simulink model "ABS_CHO"  (R2023a)
settings: Solver=ode45  StartTime=0  StopTime=15  FixedStep=0.001  RelTol=1e-3  AbsTol=1e-6
libraries: simulink x19, dspsigops x7, Solver_SF x1
(part 1 of 2)
settings Model: ExtModeTrigMode=oneshot  Creator=jhu  LastModifiedBy=USER
settings SolverCC: AutoScaleAbsTol=off  AlgebraicLoopSolver=TrustRegion
settings DataIOCC: SaveFormat=Array  SignalLoggingSaveFormat=ModelDataLogs  ReturnWorkspaceOutputs=off  SignalLoggingName=sigsOut
settings OptimizationCC: BlockReduction=off  BooleanDataType=off  ExpressionDepthLimit=2147483647  LifeSpan=inf
settings DebuggingCC: SaveWithParameterizedLinksMsg=none  UnderspecifiedInitializationDetection=Classic  MergeDetectMultiDrivingBlocksExec=none  SignalResolutionControl=TryResolveAllWithWarning  MultiTaskDSMMsg=warning  MultiTaskCondExecSysMsg=none  FcnCallInpInsideContextMsg=warning  UnconnectedInputMsg=warning  UnconnectedOutputMsg=warning  UnconnectedLineMsg=warning  StateNameClashWarn=warning  SFUnexpectedBacktrackingDiag=warning  SFNoUnconditionalDefaultTransitionDiag=warning  SFExecutionAtInitializationDiag=none  ArithmeticOperatorsInVariantConditions=warning
settings HardwareCC: ProdBitPerPointer=32  ProdBitPerSizeT=32  ProdBitPerPtrDiffT=32  ProdLargestAtomicFloat=None  ProdIntDivRoundTo=Undefined  ProdEndianess=Unspecified  ProdWordSize=32  ProdHWDeviceType=32-bit Generic  TargetUnknown=on
settings ModelReferenceCC: PropagateSignalLabelsOutOfModel=off
settings SFSimCC: SimUseLocalCustomCode=off  CustomCodeUndefinedFunction=UseInterfaceOnly
settings RTWCC: TemplateMakefile=grt_vc.tmf  RTWUseLocalCustomCode=off
settings CodeAppCC: StateflowObjectComments=on
settings GRTTargetCC: TargetFcnLib=ansi_tfl_tmw.mat  TargetLangStandard=C89/C90 (ANSI)  CombineOutputUpdateFcns=off  GRTInterface=on
settings ConfigComp: CovMetricSettings=dw  CovSaveCumulativeToWorkspaceVar=on  CovSaveSingleToWorkspaceVar=on  CovExternalEMLEnable=off

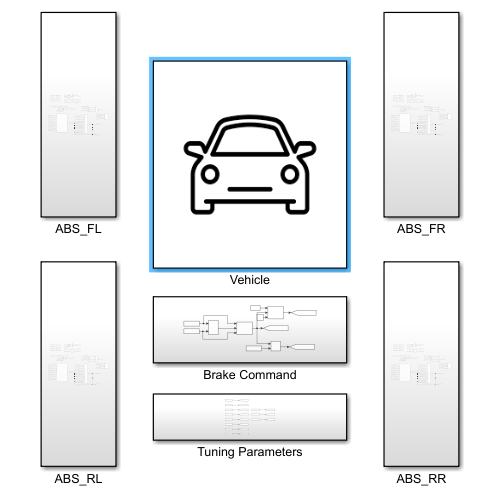
[thumbnail: Simulink's stored preview of the top-level diagram]
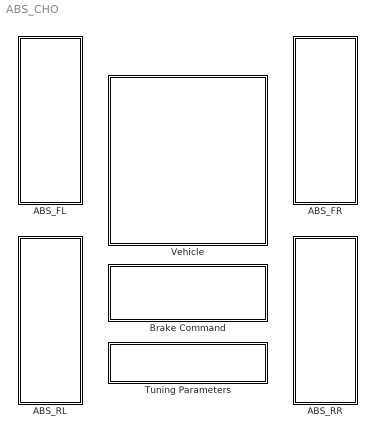
== system ABS_CHO ==
  ABS_FL : Subsystem
  ABS_FR : Subsystem
  ABS_RL : Subsystem
  ABS_RR : Subsystem
  Brake Command : Subsystem
  Tuning Parameters : Subsystem
  Vehicle : Subsystem
      mask Display: image('C:\Users\USER\Downloads\vehicle_icon.png'); % Use "Edit Image" on toolstrip to change.

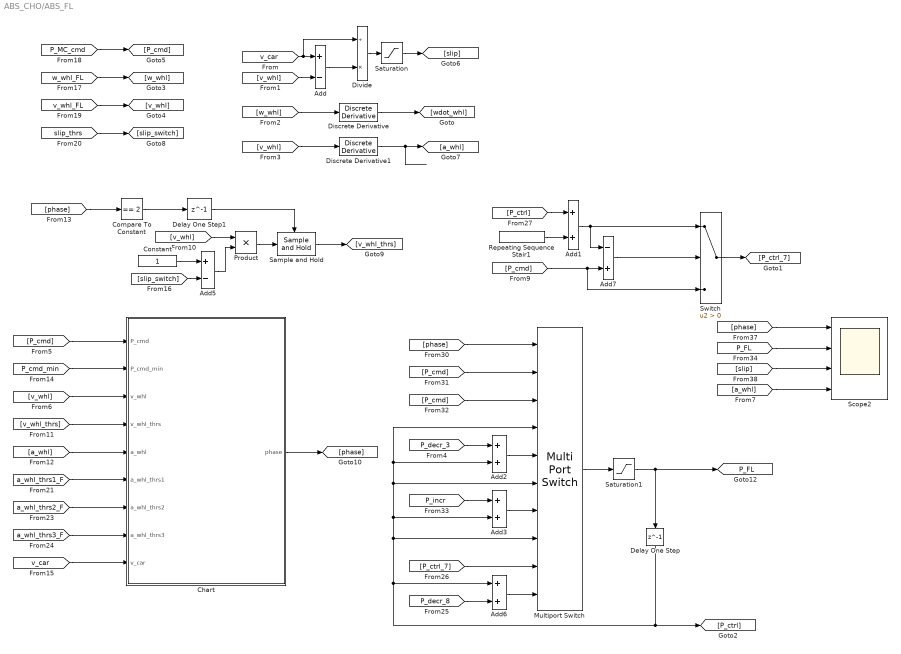
== system ABS_CHO/ABS_FL ==
  Add : Sum  Inputs=+-
  Add{1..3,6} (4 alike) : Sum
  Add5 : Sum  Inputs=+-
  Add7 : Sum  Inputs=-+
  Chart : Stateflow chart  TreatAsAtomicUnit=on
      settings: PortSchema="{\"entries\":[{\"content\":{\"sides\":[{\"content\":{\"connectorIds\":[\"In4\",\"In5\",\"In2\",\"In9\",\"In1\",\"In6\",\"In7\",\"In8\",\"In3\"]},\"type\":\"ConnectorPlacement.EquallySpacedRectSide\",\"uuid\":\"d1b40d47-5080-4bdb-9b64-2db0b8a6d570\"},{\"content\":{\"connectorIds\":[\"Out1\"],\"side\":\"RIGHT\"},\"type\":\"ConnectorPlacement.EquallySpacedRectSide\",\"uuid\":\"3562d231-244b-4945-a90c-51a654d62f0f\"},{\"content\":{\"side\":\"TOP\"},\"type\":\"ConnectorPlacement.EquallySpacedRectSide\",\"uuid\":\"6c914ffe-04dc-4ab2-bade-76d69248353c\"}]},\"type\":\"ConnectorPlacement.EquallySpacedConnector\",\"uuid\":\"36a59ec9-6bc3-461d-a020-c1da85e3b47f\"}],\"packageUris\":[\"http://schema.mathworks.com/mf0/Connector/R2020b\"],\"version\":\"1.0\"}"
  Compare To Constant : simulink/Logic and Bit Operations/Compare To Constant  relop===  const=2  OutDataTypeStr=boolean
  Constant : Constant
  Delay One Step : Delay  DelayLength=1  SampleTime=0.01
  Delay One Step1 : Delay  DelayLength=1  SampleTime=0.01
  Discrete Derivative : simulink/Discrete/Discrete Derivative  gainval=1.0  ICPrevScaledInput=0.0  OutMin=[]  OutMax=[]  OutDataType=fixdt(1, 16)  OutScaling=2^-10  DoSatur=off
  Discrete Derivative1 : simulink/Discrete/Discrete Derivative  gainval=1.0  ICPrevScaledInput=0.0  OutMin=[]  OutMax=[]  OutDataType=fixdt(1, 16)  OutScaling=2^-10  DoSatur=off
  Divide : Product  Inputs=/*
  Multiport Switch : MultiPortSwitch  DataPortOrder=Zero-based contiguous  Inputs=9  zeroidx=on  SaturateOnIntegerOverflow=off  InputSameDT=off
  Product : Product
  Repeating Sequence Stair1 : simulink/Sources/Repeating Sequence Stair  OutValues=[0.2 0].'  tsamp=0.01  OutMin=[]  OutMax=[]  OutDataTypeStr=double  OutputDataTypeScalingMode=double  OutDataType=fixdt(0,8)  ConRadixGroup=Best Precision: Vector-wise  OutScaling=2^-12
  Sample and Hold : dspsigops/Sample and Hold  trig=Rising edge  initCond=0  latchinput=off
  Saturation : Saturate  UpperLimit=1  LowerLimit=-1
  Saturation1 : Saturate  UpperLimit=30  LowerLimit=0
  Scope2 : Scope  NumInputPorts=4
  Switch : Switch  Criteria=u2 > Threshold  SaturateOnIntegerOverflow=off  InputSameDT=off
  tag scope: P_FL=global
  wires:
  Delay One Step/1 -> [P_ctrl], Add6/1, Multiport Switch/6, Add2/2, Multiport Switch/4, Add3/2, Multiport Switch/8
  Switch/1 -> [P_ctrl_7]
  Add7/1 -> Switch/2
  [P_cmd] -> Add7/2, Switch/3
  Add1/1 -> Add7/1, Switch/1
  Repeating Sequence Stair1/1 -> Add1/2
  [P_ctrl] -> Add1/1
  [v_car] -> Divide/1, Add/1
  [v_whl] -> Add/2
  Add/1 -> Divide/2
  Divide/1 -> Saturation/1
  Saturation/1 -> [slip]
  [w_whl] -> Discrete Derivative/1
  Discrete Derivative/1 -> [wdot_whl]
  [v_whl] -> Discrete Derivative1/1
  Discrete Derivative1/1 -> [a_whl]
  [slip_thrs] -> [slip_switch]
  [v_whl] -> Product/1
  Sample and Hold/1 -> [v_whl_thrs]
  Chart/1(phase) -> [phase]
  [w_whl_FL] -> [w_whl]
  [v_whl_FL] -> [v_whl]
  [P_MC_cmd] -> [P_cmd]
  [phase] -> Multiport Switch/1
  [P_cmd] -> Multiport Switch/2
  [P_cmd] -> Multiport Switch/3
  Multiport Switch/1 -> Saturation1/1
  Add2/1 -> Multiport Switch/5
  [P_decr_3] -> Add2/1
  Add3/1 -> Multiport Switch/7
  [P_ctrl_7] -> Multiport Switch/9
  Saturation1/1 -> Delay One Step/1, [P_FL]
  [P_incr] -> Add3/1
  Constant/1 -> Add5/1
  [slip_switch] -> Add5/2
  Add5/1 -> Product/2
  Product/1 -> Sample and Hold/1
  [phase] -> Scope2/1
  [P_FL] -> Scope2/2
  [slip] -> Scope2/3
  [P_cmd] -> Chart/4(P_cmd)
  [P_cmd_min] -> Chart/5(P_cmd_min)
  [v_whl] -> Chart/2(v_whl)
  [v_whl_thrs] -> Chart/9(v_whl_thrs)
  [a_whl] -> Chart/1(a_whl)
  [v_car] -> Chart/3(v_car)
  [a_whl] -> Scope2/4
  [phase] -> Compare To Constant/1
  Compare To Constant/1 -> Delay One Step1/1
  Delay One Step1/1 -> Sample and Hold/Trigger
  [a_whl_thrs1_F] -> Chart/6(a_whl_thrs1)
  [a_whl_thrs2_F] -> Chart/7(a_whl_thrs2)
  [a_whl_thrs3_F] -> Chart/8(a_whl_thrs3)
  Add6/1 -> Multiport Switch/10
  [P_decr_8] -> Add6/2

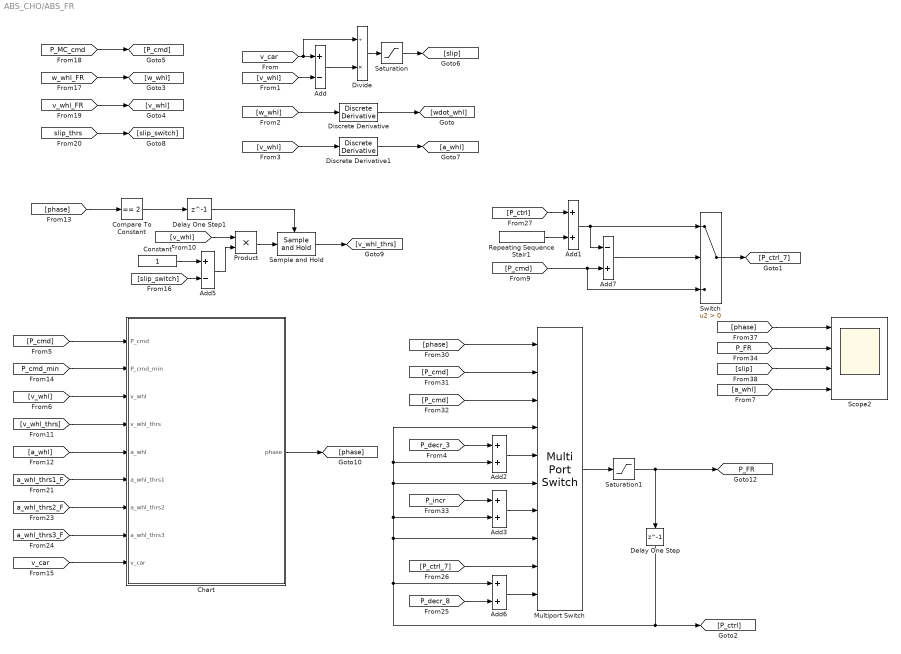
== system ABS_CHO/ABS_FR ==
  Add : Sum  Inputs=+-
  Add{1..3,6} (4 alike) : Sum
  Add5 : Sum  Inputs=+-
  Add7 : Sum  Inputs=-+
  Chart : Stateflow chart  TreatAsAtomicUnit=on
      settings: PortSchema="{\"entries\":[{\"content\":{\"sides\":[{\"content\":{\"connectorIds\":[\"In4\",\"In5\",\"In2\",\"In9\",\"In1\",\"In6\",\"In7\",\"In8\",\"In3\"]},\"type\":\"ConnectorPlacement.EquallySpacedRectSide\",\"uuid\":\"d1b40d47-5080-4bdb-9b64-2db0b8a6d570\"},{\"content\":{\"connectorIds\":[\"Out1\"],\"side\":\"RIGHT\"},\"type\":\"ConnectorPlacement.EquallySpacedRectSide\",\"uuid\":\"3562d231-244b-4945-a90c-51a654d62f0f\"},{\"content\":{\"side\":\"TOP\"},\"type\":\"ConnectorPlacement.EquallySpacedRectSide\",\"uuid\":\"6c914ffe-04dc-4ab2-bade-76d69248353c\"}]},\"type\":\"ConnectorPlacement.EquallySpacedConnector\",\"uuid\":\"36a59ec9-6bc3-461d-a020-c1da85e3b47f\"}],\"packageUris\":[\"http://schema.mathworks.com/mf0/Connector/R2020b\"],\"version\":\"1.0\"}"
  Compare To Constant : simulink/Logic and Bit Operations/Compare To Constant  relop===  const=2  OutDataTypeStr=boolean
  Constant : Constant
  Delay One Step : Delay  DelayLength=1  SampleTime=0.01
  Delay One Step1 : Delay  DelayLength=1  SampleTime=0.01
  Discrete Derivative : simulink/Discrete/Discrete Derivative  gainval=1.0  ICPrevScaledInput=0.0  OutMin=[]  OutMax=[]  OutDataType=fixdt(1, 16)  OutScaling=2^-10  DoSatur=off
  Discrete Derivative1 : simulink/Discrete/Discrete Derivative  gainval=1.0  ICPrevScaledInput=0.0  OutMin=[]  OutMax=[]  OutDataType=fixdt(1, 16)  OutScaling=2^-10  DoSatur=off
  Divide : Product  Inputs=/*
  Multiport Switch : MultiPortSwitch  DataPortOrder=Zero-based contiguous  Inputs=9  zeroidx=on  SaturateOnIntegerOverflow=off  InputSameDT=off
  Product : Product
  Repeating Sequence Stair1 : simulink/Sources/Repeating Sequence Stair  OutValues=[0.2 0].'  tsamp=0.01  OutMin=[]  OutMax=[]  OutDataTypeStr=double  OutputDataTypeScalingMode=double  OutDataType=fixdt(0,8)  ConRadixGroup=Best Precision: Vector-wise  OutScaling=2^-12
  Sample and Hold : dspsigops/Sample and Hold  trig=Rising edge  initCond=0  latchinput=off
  Saturation : Saturate  UpperLimit=1  LowerLimit=-1
  Saturation1 : Saturate  UpperLimit=30  LowerLimit=0
  Scope2 : Scope  NumInputPorts=4
  Switch : Switch  Criteria=u2 > Threshold  SaturateOnIntegerOverflow=off  InputSameDT=off
  tag scope: P_FR=global
  wires:
  [P_decr_8] -> Add6/2
  Add6/1 -> Multiport Switch/10
  [a_whl_thrs3_F] -> Chart/8(a_whl_thrs3)
  [a_whl_thrs2_F] -> Chart/7(a_whl_thrs2)
  [a_whl_thrs1_F] -> Chart/6(a_whl_thrs1)
  Delay One Step1/1 -> Sample and Hold/Trigger
  Compare To Constant/1 -> Delay One Step1/1
  [phase] -> Compare To Constant/1
  [a_whl] -> Scope2/4
  [v_car] -> Chart/3(v_car)
  [a_whl] -> Chart/1(a_whl)
  [v_whl_thrs] -> Chart/9(v_whl_thrs)
  [v_whl] -> Chart/2(v_whl)
  [P_cmd_min] -> Chart/5(P_cmd_min)
  [P_cmd] -> Chart/4(P_cmd)
  [slip] -> Scope2/3
  [P_FR] -> Scope2/2
  [phase] -> Scope2/1
  Product/1 -> Sample and Hold/1
  Add5/1 -> Product/2
  [slip_switch] -> Add5/2
  Constant/1 -> Add5/1
  [P_incr] -> Add3/1
  Saturation1/1 -> [P_FR], Delay One Step/1
  [P_ctrl_7] -> Multiport Switch/9
  Add3/1 -> Multiport Switch/7
  [P_decr_3] -> Add2/1
  Add2/1 -> Multiport Switch/5
  Multiport Switch/1 -> Saturation1/1
  [P_cmd] -> Multiport Switch/3
  [P_cmd] -> Multiport Switch/2
  [phase] -> Multiport Switch/1
  [P_MC_cmd] -> [P_cmd]
  [v_whl_FR] -> [v_whl]
  [w_whl_FR] -> [w_whl]
  Chart/1(phase) -> [phase]
  Sample and Hold/1 -> [v_whl_thrs]
  [v_whl] -> Product/1
  [slip_thrs] -> [slip_switch]
  Discrete Derivative1/1 -> [a_whl]
  [v_whl] -> Discrete Derivative1/1
  Discrete Derivative/1 -> [wdot_whl]
  [w_whl] -> Discrete Derivative/1
  Saturation/1 -> [slip]
  Divide/1 -> Saturation/1
  Add/1 -> Divide/2
  [v_whl] -> Add/2
  [v_car] -> Add/1, Divide/1
  [P_ctrl] -> Add1/1
  Repeating Sequence Stair1/1 -> Add1/2
  Add1/1 -> Switch/1, Add7/1
  [P_cmd] -> Switch/3, Add7/2
  Add7/1 -> Switch/2
  Switch/1 -> [P_ctrl_7]
  Delay One Step/1 -> Multiport Switch/8, Add3/2, Multiport Switch/4, Add2/2, Multiport Switch/6, Add6/1, [P_ctrl]

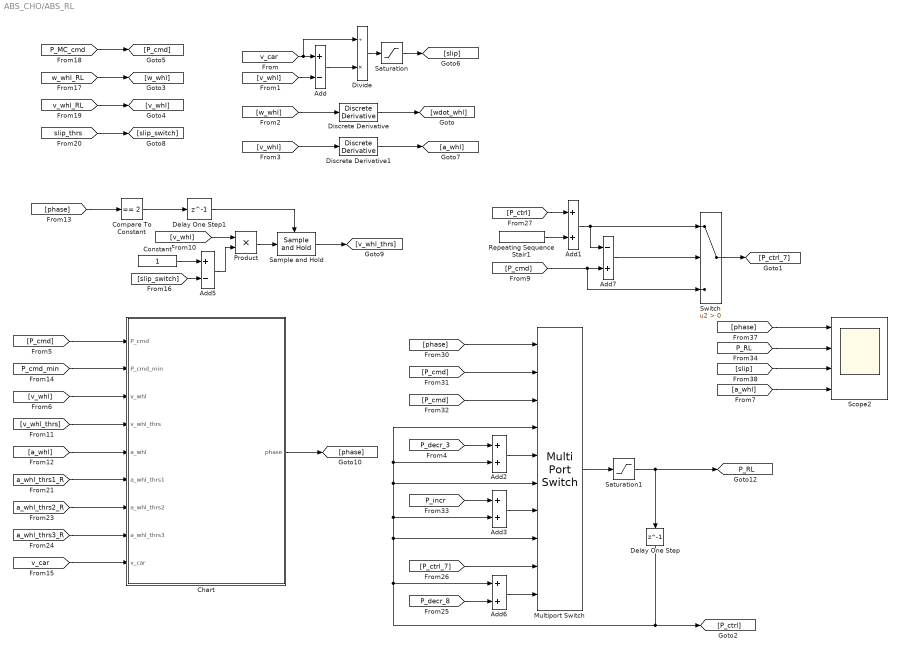
== system ABS_CHO/ABS_RL ==
  Add : Sum  Inputs=+-
  Add{1..3,6} (4 alike) : Sum
  Add5 : Sum  Inputs=+-
  Add7 : Sum  Inputs=-+
  Chart : Stateflow chart  TreatAsAtomicUnit=on
      settings: PortSchema="{\"entries\":[{\"content\":{\"sides\":[{\"content\":{\"connectorIds\":[\"In4\",\"In5\",\"In2\",\"In9\",\"In1\",\"In6\",\"In7\",\"In8\",\"In3\"]},\"type\":\"ConnectorPlacement.EquallySpacedRectSide\",\"uuid\":\"d1b40d47-5080-4bdb-9b64-2db0b8a6d570\"},{\"content\":{\"connectorIds\":[\"Out1\"],\"side\":\"RIGHT\"},\"type\":\"ConnectorPlacement.EquallySpacedRectSide\",\"uuid\":\"3562d231-244b-4945-a90c-51a654d62f0f\"},{\"content\":{\"side\":\"TOP\"},\"type\":\"ConnectorPlacement.EquallySpacedRectSide\",\"uuid\":\"6c914ffe-04dc-4ab2-bade-76d69248353c\"}]},\"type\":\"ConnectorPlacement.EquallySpacedConnector\",\"uuid\":\"36a59ec9-6bc3-461d-a020-c1da85e3b47f\"}],\"packageUris\":[\"http://schema.mathworks.com/mf0/Connector/R2020b\"],\"version\":\"1.0\"}"
  Compare To Constant : simulink/Logic and Bit Operations/Compare To Constant  relop===  const=2  OutDataTypeStr=boolean
  Constant : Constant
  Delay One Step : Delay  DelayLength=1  SampleTime=0.01
  Delay One Step1 : Delay  DelayLength=1  SampleTime=0.01
  Discrete Derivative : simulink/Discrete/Discrete Derivative  gainval=1.0  ICPrevScaledInput=0.0  OutMin=[]  OutMax=[]  OutDataType=fixdt(1, 16)  OutScaling=2^-10  DoSatur=off
  Discrete Derivative1 : simulink/Discrete/Discrete Derivative  gainval=1.0  ICPrevScaledInput=0.0  OutMin=[]  OutMax=[]  OutDataType=fixdt(1, 16)  OutScaling=2^-10  DoSatur=off
  Divide : Product  Inputs=/*
  Multiport Switch : MultiPortSwitch  DataPortOrder=Zero-based contiguous  Inputs=9  zeroidx=on  SaturateOnIntegerOverflow=off  InputSameDT=off
  Product : Product
  Repeating Sequence Stair1 : simulink/Sources/Repeating Sequence Stair  OutValues=[0.2 0].'  tsamp=0.01  OutMin=[]  OutMax=[]  OutDataTypeStr=double  OutputDataTypeScalingMode=double  OutDataType=fixdt(0,8)  ConRadixGroup=Best Precision: Vector-wise  OutScaling=2^-12
  Sample and Hold : dspsigops/Sample and Hold  trig=Rising edge  initCond=0  latchinput=off
  Saturation : Saturate  UpperLimit=1  LowerLimit=-1
  Saturation1 : Saturate  UpperLimit=30  LowerLimit=0
  Scope2 : Scope  NumInputPorts=4
  Switch : Switch  Criteria=u2 > Threshold  SaturateOnIntegerOverflow=off  InputSameDT=off
  tag scope: P_RL=global
  wires:
  Delay One Step/1 -> [P_ctrl], Add6/1, Multiport Switch/6, Add2/2, Multiport Switch/4, Add3/2, Multiport Switch/8
  Switch/1 -> [P_ctrl_7]
  Add7/1 -> Switch/2
  [P_cmd] -> Add7/2, Switch/3
  Add1/1 -> Add7/1, Switch/1
  Repeating Sequence Stair1/1 -> Add1/2
  [P_ctrl] -> Add1/1
  [v_car] -> Divide/1, Add/1
  [v_whl] -> Add/2
  Add/1 -> Divide/2
  Divide/1 -> Saturation/1
  Saturation/1 -> [slip]
  [w_whl] -> Discrete Derivative/1
  Discrete Derivative/1 -> [wdot_whl]
  [v_whl] -> Discrete Derivative1/1
  Discrete Derivative1/1 -> [a_whl]
  [slip_thrs] -> [slip_switch]
  [v_whl] -> Product/1
  Sample and Hold/1 -> [v_whl_thrs]
  Chart/1(phase) -> [phase]
  [w_whl_RL] -> [w_whl]
  [v_whl_RL] -> [v_whl]
  [P_MC_cmd] -> [P_cmd]
  [phase] -> Multiport Switch/1
  [P_cmd] -> Multiport Switch/2
  [P_cmd] -> Multiport Switch/3
  Multiport Switch/1 -> Saturation1/1
  Add2/1 -> Multiport Switch/5
  [P_decr_3] -> Add2/1
  Add3/1 -> Multiport Switch/7
  [P_ctrl_7] -> Multiport Switch/9
  Saturation1/1 -> Delay One Step/1, [P_RL]
  [P_incr] -> Add3/1
  Constant/1 -> Add5/1
  [slip_switch] -> Add5/2
  Add5/1 -> Product/2
  Product/1 -> Sample and Hold/1
  [phase] -> Scope2/1
  [P_RL] -> Scope2/2
  [slip] -> Scope2/3
  [P_cmd] -> Chart/4(P_cmd)
  [P_cmd_min] -> Chart/5(P_cmd_min)
  [v_whl] -> Chart/2(v_whl)
  [v_whl_thrs] -> Chart/9(v_whl_thrs)
  [a_whl] -> Chart/1(a_whl)
  [v_car] -> Chart/3(v_car)
  [a_whl] -> Scope2/4
  [phase] -> Compare To Constant/1
  Compare To Constant/1 -> Delay One Step1/1
  Delay One Step1/1 -> Sample and Hold/Trigger
  [a_whl_thrs1_R] -> Chart/6(a_whl_thrs1)
  [a_whl_thrs2_R] -> Chart/7(a_whl_thrs2)
  [a_whl_thrs3_R] -> Chart/8(a_whl_thrs3)
  Add6/1 -> Multiport Switch/10
  [P_decr_8] -> Add6/2

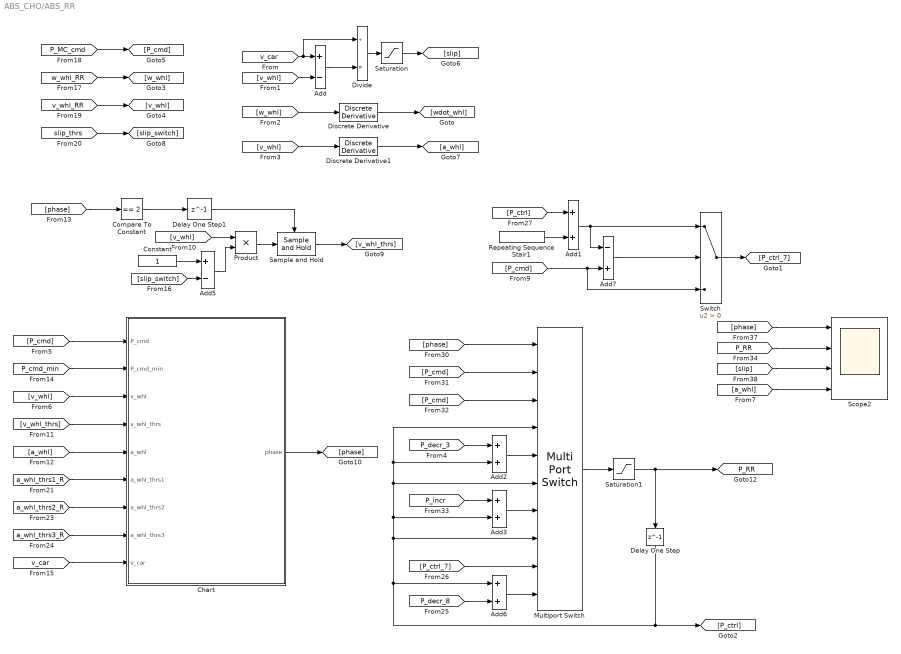
== system ABS_CHO/ABS_RR ==
  Add : Sum  Inputs=+-
  Add{1..3,6} (4 alike) : Sum
  Add5 : Sum  Inputs=+-
  Add7 : Sum  Inputs=-+
  Chart : Stateflow chart  TreatAsAtomicUnit=on
      settings: PortSchema="{\"entries\":[{\"content\":{\"sides\":[{\"content\":{\"connectorIds\":[\"In4\",\"In5\",\"In2\",\"In9\",\"In1\",\"In6\",\"In7\",\"In8\",\"In3\"]},\"type\":\"ConnectorPlacement.EquallySpacedRectSide\",\"uuid\":\"d1b40d47-5080-4bdb-9b64-2db0b8a6d570\"},{\"content\":{\"connectorIds\":[\"Out1\"],\"side\":\"RIGHT\"},\"type\":\"ConnectorPlacement.EquallySpacedRectSide\",\"uuid\":\"3562d231-244b-4945-a90c-51a654d62f0f\"},{\"content\":{\"side\":\"TOP\"},\"type\":\"ConnectorPlacement.EquallySpacedRectSide\",\"uuid\":\"6c914ffe-04dc-4ab2-bade-76d69248353c\"}]},\"type\":\"ConnectorPlacement.EquallySpacedConnector\",\"uuid\":\"36a59ec9-6bc3-461d-a020-c1da85e3b47f\"}],\"packageUris\":[\"http://schema.mathworks.com/mf0/Connector/R2020b\"],\"version\":\"1.0\"}"
  Compare To Constant : simulink/Logic and Bit Operations/Compare To Constant  relop===  const=2  OutDataTypeStr=boolean
  Constant : Constant
  Delay One Step : Delay  DelayLength=1  SampleTime=0.01
  Delay One Step1 : Delay  DelayLength=1  SampleTime=0.01
  Discrete Derivative : simulink/Discrete/Discrete Derivative  gainval=1.0  ICPrevScaledInput=0.0  OutMin=[]  OutMax=[]  OutDataType=fixdt(1, 16)  OutScaling=2^-10  DoSatur=off
  Discrete Derivative1 : simulink/Discrete/Discrete Derivative  gainval=1.0  ICPrevScaledInput=0.0  OutMin=[]  OutMax=[]  OutDataType=fixdt(1, 16)  OutScaling=2^-10  DoSatur=off
  Divide : Product  Inputs=/*
  Multiport Switch : MultiPortSwitch  DataPortOrder=Zero-based contiguous  Inputs=9  zeroidx=on  SaturateOnIntegerOverflow=off  InputSameDT=off
  Product : Product
  Repeating Sequence Stair1 : simulink/Sources/Repeating Sequence Stair  OutValues=[0.2 0].'  tsamp=0.01  OutMin=[]  OutMax=[]  OutDataTypeStr=double  OutputDataTypeScalingMode=double  OutDataType=fixdt(0,8)  ConRadixGroup=Best Precision: Vector-wise  OutScaling=2^-12
  Sample and Hold : dspsigops/Sample and Hold  trig=Rising edge  initCond=0  latchinput=off
  Saturation : Saturate  UpperLimit=1  LowerLimit=-1
  Saturation1 : Saturate  UpperLimit=30  LowerLimit=0
  Scope2 : Scope  NumInputPorts=4
  Switch : Switch  Criteria=u2 > Threshold  SaturateOnIntegerOverflow=off  InputSameDT=off
  tag scope: P_RR=global
  wires:
  Delay One Step/1 -> [P_ctrl], Add6/1, Multiport Switch/6, Add2/2, Multiport Switch/4, Add3/2, Multiport Switch/8
  Switch/1 -> [P_ctrl_7]
  Add7/1 -> Switch/2
  [P_cmd] -> Add7/2, Switch/3
  Add1/1 -> Add7/1, Switch/1
  Repeating Sequence Stair1/1 -> Add1/2
  [P_ctrl] -> Add1/1
  [v_car] -> Divide/1, Add/1
  [v_whl] -> Add/2
  Add/1 -> Divide/2
  Divide/1 -> Saturation/1
  Saturation/1 -> [slip]
  [w_whl] -> Discrete Derivative/1
  Discrete Derivative/1 -> [wdot_whl]
  [v_whl] -> Discrete Derivative1/1
  Discrete Derivative1/1 -> [a_whl]
  [slip_thrs] -> [slip_switch]
  [v_whl] -> Product/1
  Sample and Hold/1 -> [v_whl_thrs]
  Chart/1(phase) -> [phase]
  [w_whl_RR] -> [w_whl]
  [v_whl_RR] -> [v_whl]
  [P_MC_cmd] -> [P_cmd]
  [phase] -> Multiport Switch/1
  [P_cmd] -> Multiport Switch/2
  [P_cmd] -> Multiport Switch/3
  Multiport Switch/1 -> Saturation1/1
  Add2/1 -> Multiport Switch/5
  [P_decr_3] -> Add2/1
  Add3/1 -> Multiport Switch/7
  [P_ctrl_7] -> Multiport Switch/9
  Saturation1/1 -> Delay One Step/1, [P_RR]
  [P_incr] -> Add3/1
  Constant/1 -> Add5/1
  [slip_switch] -> Add5/2
  Add5/1 -> Product/2
  Product/1 -> Sample and Hold/1
  [phase] -> Scope2/1
  [P_RR] -> Scope2/2
  [slip] -> Scope2/3
  [P_cmd] -> Chart/4(P_cmd)
  [P_cmd_min] -> Chart/5(P_cmd_min)
  [v_whl] -> Chart/2(v_whl)
  [v_whl_thrs] -> Chart/9(v_whl_thrs)
  [a_whl] -> Chart/1(a_whl)
  [v_car] -> Chart/3(v_car)
  [a_whl] -> Scope2/4
  [phase] -> Compare To Constant/1
  Compare To Constant/1 -> Delay One Step1/1
  Delay One Step1/1 -> Sample and Hold/Trigger
  [a_whl_thrs1_R] -> Chart/6(a_whl_thrs1)
  [a_whl_thrs2_R] -> Chart/7(a_whl_thrs2)
  [a_whl_thrs3_R] -> Chart/8(a_whl_thrs3)
  Add6/1 -> Multiport Switch/10
  [P_decr_8] -> Add6/2

== system ABS_CHO/Brake Command ==
  Add : Sum  Inputs=-+
  Constant : Constant
  Ground : Ground
  P_cmd : Constant  Value=5  SampleTime=0.01
  P_cmd1 : Constant  Value=100  SampleTime=0.01
  Product : Product
  Ramp : simulink/Sources/Ramp  slope=20  start=5  InitialOutput=0
  Switch : Switch  Criteria=u2 > Threshold  SaturateOnIntegerOverflow=off  InputSameDT=off
  Switch1 : Switch  Criteria=u2 > Threshold  SaturateOnIntegerOverflow=off  InputSameDT=off
  tag scope: P_MC_cmd=global, brk_stat=global, brk_tq_cmd=global
  wires:
  P_cmd/1 -> Switch/3, Add/2
  Ramp/1 -> Switch/1, Add/1
  Add/1 -> Switch/2
  Switch/1 -> Product/1, Switch1/2, [P_MC_cmd]
  Constant/1 -> Switch1/1
  Ground/1 -> Switch1/3
  Switch1/1 -> [brk_stat]
  P_cmd1/1 -> Product/2
  Product/1 -> [brk_tq_cmd]

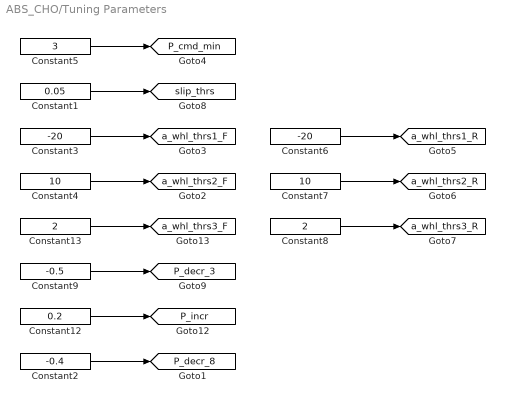
== system ABS_CHO/Tuning Parameters ==
  Constant1 : Constant  Value=0.05  SampleTime=0.01
  Constant12 : Constant  Value=0.2  SampleTime=0.01
  Constant13 : Constant  Value=2  SampleTime=0.01
  Constant2 : Constant  Value=-0.4  SampleTime=0.01
  Constant3 : Constant  Value=-20  SampleTime=0.01
  Constant4 : Constant  Value=10  SampleTime=0.01
  Constant5 : Constant  Value=3  SampleTime=0.01
  Constant6 : Constant  Value=-20  SampleTime=0.01
  Constant7 : Constant  Value=10  SampleTime=0.01
  Constant8 : Constant  Value=2  SampleTime=0.01
  Constant9 : Constant  Value=-0.5  SampleTime=0.01
  tag scope: P_cmd_min=global, P_decr_3=global, P_decr_8=global, P_incr=global, a_whl_thrs1_F=global, a_whl_thrs1_R=global, a_whl_thrs2_F=global, a_whl_thrs2_R=global, a_whl_thrs3_F=global, a_whl_thrs3_R=global, slip_thrs=global
  wires:
  Constant1/1 -> [slip_thrs]
  Constant4/1 -> [a_whl_thrs2_F]
  Constant3/1 -> [a_whl_thrs1_F]
  Constant5/1 -> [P_cmd_min]
  Constant9/1 -> [P_decr_3]
  Constant12/1 -> [P_incr]
  Constant13/1 -> [a_whl_thrs3_F]
  Constant2/1 -> [P_decr_8]
  Constant6/1 -> [a_whl_thrs1_R]
  Constant7/1 -> [a_whl_thrs2_R]
  Constant8/1 -> [a_whl_thrs3_R]

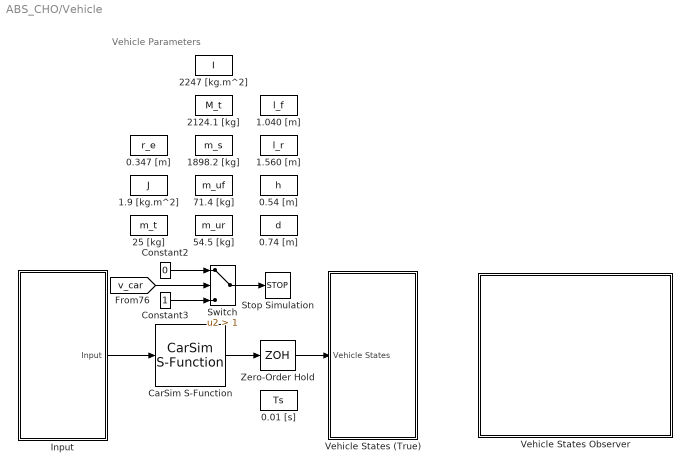
== system ABS_CHO/Vehicle ==
  note: Vehicle Parameters
  0.01 [s] : DataStoreMemory  DataStoreName=Ts  WriteAfterWriteMsg=warning  InitialValue=0.01  ShowAdditionalParam=off  OutDataTypeStr=double
  0.347 [m] : DataStoreMemory  DataStoreName=r_e  WriteAfterWriteMsg=warning  InitialValue=0.287  ShowAdditionalParam=off  OutDataTypeStr=double
  0.54 [m] : DataStoreMemory  DataStoreName=h  WriteAfterWriteMsg=warning  InitialValue=0.54  ShowAdditionalParam=off  OutDataTypeStr=double
  0.74 [m] : DataStoreMemory  DataStoreName=d  WriteAfterWriteMsg=warning  InitialValue=0.74  ShowAdditionalParam=off  OutDataTypeStr=double
  1.040 [m] : DataStoreMemory  DataStoreName=l_f  WriteAfterWriteMsg=warning  InitialValue=1.040  ShowAdditionalParam=off  OutDataTypeStr=double
  1.560 [m] : DataStoreMemory  DataStoreName=l_r  WriteAfterWriteMsg=warning  InitialValue=1.560  ShowAdditionalParam=off  OutDataTypeStr=double
  1.9 [kg.m^2] : DataStoreMemory  DataStoreName=J  WriteAfterWriteMsg=warning  InitialValue=0.8  ShowAdditionalParam=off  OutDataTypeStr=double
  1898.2 [kg] : DataStoreMemory  DataStoreName=m_s  WriteAfterWriteMsg=warning  InitialValue=1134  ShowAdditionalParam=off  OutDataTypeStr=double
  2124.1 [kg] : DataStoreMemory  DataStoreName=M_t  WriteAfterWriteMsg=warning  InitialValue=1323.9  ShowAdditionalParam=off  OutDataTypeStr=double
  2247 [kg.m^2] : DataStoreMemory  DataStoreName=I  WriteAfterWriteMsg=warning  InitialValue=1343.1  ShowAdditionalParam=off  OutDataTypeStr=double
  25 [kg] : DataStoreMemory  DataStoreName=m_t  WriteAfterWriteMsg=warning  InitialValue=16  ShowAdditionalParam=off  OutDataTypeStr=double
  54.5 [kg] : DataStoreMemory  DataStoreName=m_ur  WriteAfterWriteMsg=warning  InitialValue=54.5  ShowAdditionalParam=off  OutDataTypeStr=double
  71.4 [kg] : DataStoreMemory  DataStoreName=m_uf  WriteAfterWriteMsg=warning  InitialValue=71.4  ShowAdditionalParam=off  OutDataTypeStr=double
  CarSim S-Function : Solver_SF/CarSim S-Function  Priority=1  SIMFILE=simfile.sim  Run_RTs=off  vs_state_ind=Run  StopMode_ind=Vehicle Model
  Constant2 : Constant  Value=0
  Constant3 : Constant
  Input : Subsystem
  Stop Simulation : Stop
  Switch : Switch  Criteria=u2 > Threshold  Threshold=1  SaturateOnIntegerOverflow=off  InputSameDT=off
  Vehicle States (True) : Subsystem
  Vehicle States Observer : Subsystem
  Zero-Order Hold : ZeroOrderHold  SampleTime=0.01
  wires:
  CarSim S-Function/1 -> Zero-Order Hold/1
  Zero-Order Hold/1 -> Vehicle States (True)/1(Vehicle States)
  Input/1(Input) -> CarSim S-Function/1
  Constant2/1 -> Switch/1
  [v_car] -> Switch/2
  Constant3/1 -> Switch/3
  Switch/1 -> Stop Simulation/1

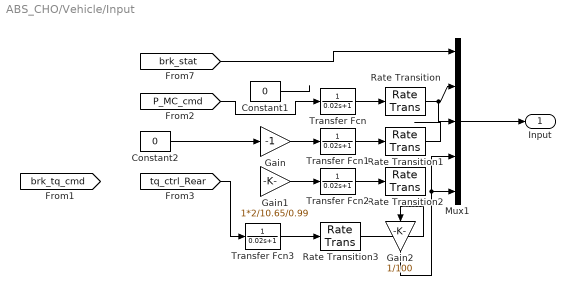
== system ABS_CHO/Vehicle/Input ==
  Constant1 : Constant  Value=0
  Constant2 : Constant  Value=0
  Gain : Gain  Gain=-1
  Gain1 : Gain  Gain=1*2/10.65/0.99
  Gain2 : Gain  Gain=1/100
  Mux1 : Mux  Inputs=5
  Rate Transition{,1..3} (4 alike) : RateTransition  OutPortSampleTime=0.01
  Transfer Fcn{,1..3} (4 alike) : TransferFcn  Denominator=[0.02 1]
  Input : Outport
  wires:
  Rate Transition1/1 -> ?
  Transfer Fcn/1 -> Rate Transition/1
  Transfer Fcn1/1 -> Rate Transition1/1
  Rate Transition/1 -> Mux1/3, Mux1/2
  [P_MC_cmd] -> Transfer Fcn/1
  Mux1/1 -> Input/1
  [brk_stat] -> Mux1/1
  Constant2/1 -> Gain/1
  Transfer Fcn2/1 -> Rate Transition2/1
  Gain/1 -> Transfer Fcn1/1
  Gain1/1 -> Transfer Fcn2/1
  Gain2/1 -> Mux1/5, Mux1/4
  Transfer Fcn3/1 -> Rate Transition3/1
  Rate Transition3/1 -> Gain2/1
  [tq_ctrl_Rear] -> Transfer Fcn3/1
  Constant1/1 -> ?

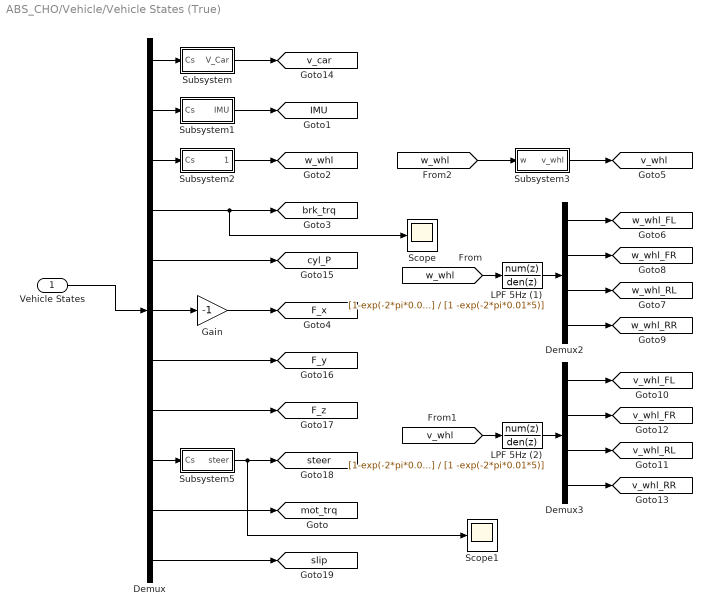
== system ABS_CHO/Vehicle/Vehicle States (True) ==
  Vehicle States : Inport
  Demux : Demux  Outputs=[1 3 4 4 4 4 4 4 4 4 4]
  Demux2 : Demux
  Demux3 : Demux
  Gain : Gain  Gain=-1
  LPF 5Hz (1) : DiscreteFilter  Numerator=[1-exp(-2*pi*0.01*5)]  Denominator=[1 -exp(-2*pi*0.01*5)]  SampleTime=0.01
  LPF 5Hz (2) : DiscreteFilter  Numerator=[1-exp(-2*pi*0.01*5)]  Denominator=[1 -exp(-2*pi*0.01*5)]  SampleTime=0.01
  Scope : Scope
  Scope1 : Scope
  Subsystem : Subsystem
  Subsystem1 : Subsystem
  Subsystem2 : Subsystem
  Subsystem3 : Subsystem
  Subsystem5 : Subsystem
  tag scope: F_x=global, F_y=global, F_z=global, IMU=global, brk_trq=global, cyl_P=global, mot_trq=global, slip=global, steer=global, v_car=global, v_whl=global, v_whl_FL=global, v_whl_FR=global, v_whl_RL=global, v_whl_RR=global, w_whl=global, w_whl_FL=global, w_whl_FR=global, w_whl_RL=global, w_whl_RR=global
  wires:
  Demux2/4 -> [w_whl_RR]
  Demux/6 -> Gain/1
  [v_whl] -> LPF 5Hz (2)/1
  Demux3/4 -> [v_whl_RR]
  Demux3/2 -> [v_whl_FR]
  Demux2/2 -> [w_whl_FR]
  [w_whl] -> LPF 5Hz (1)/1
  Demux3/1 -> [v_whl_FL]
  Demux2/3 -> [w_whl_RL]
  Demux/2 -> Subsystem1/1(Cs)
  Subsystem/1(V_Car) -> [v_car]
  Demux3/3 -> [v_whl_RL]
  LPF 5Hz (1)/1 -> Demux2/1
  Demux2/1 -> [w_whl_FL]
  Demux/1 -> Subsystem/1(Cs)
  Demux/7 -> [F_y]
  LPF 5Hz (2)/1 -> Demux3/1
  Subsystem1/1(IMU) -> [IMU]
  Vehicle States/1 -> Demux/1
  Demux/3 -> Subsystem2/1(Cs)
  Subsystem2/1(w_whl) -> [w_whl]
  Subsystem3/1(v_whl) -> [v_whl]
  [w_whl] -> Subsystem3/1(w)
  Demux/4 -> Scope/1, [brk_trq]
  Demux/5 -> [cyl_P]
  Demux/8 -> [F_z]
  Demux/10 -> [mot_trq]
  Gain/1 -> [F_x]
  Demux/11 -> [slip]
  Subsystem5/1(steer) -> Scope1/1, [steer]
  Demux/9 -> Subsystem5/1(Cs)

== system ABS_CHO/Vehicle/Vehicle States Observer ==
  Rear Wheel Torque Control : Subsystem
  "Tire Force (Fx, Fy) Estimation" : Subsystem
  Vertical Tire Force (Fz) Estimation : Subsystem

== system ABS_CHO/Vehicle/Vehicle States (True)/Subsystem ==
  note: [m/s]
  Cs : Inport
  Add1 : Sum
  Gain3 : Gain  Gain=1/3.6
  Random Number : RandomNumber  Variance=0.0005  Seed=2  SampleTime=0.01
  V_Car : Outport
  wires:
  Random Number/1 -> Add1/1
  Cs/1 -> Add1/2
  Add1/1 -> Gain3/1
  Gain3/1 -> V_Car/1

== system ABS_CHO/Vehicle/Vehicle States (True)/Subsystem1 ==
  note: long. a [m/s^2]
  note: lat. a [m/s^2]
  note: yaw rate [rad/s]
  Cs : Inport
  Add{,1..5} (6 alike) : Sum
  Demux : Demux  Outputs=3
  Gain1 : Gain  Gain=9.8
  Gain2 : Gain  Gain=pi/180
  Gain4 : Gain  Gain=9.8
  Mux : Mux  Inputs=3
  Random Number1 : RandomNumber  Variance=0.0002  Seed=2  SampleTime=0.01
  Random Number2 : RandomNumber  Variance=0.0002  Seed=1  SampleTime=0.01
  Random Number3 : RandomNumber  Variance=0.003  Seed=3  SampleTime=0.01
  Random Number4 : RandomNumber  Variance=0.001  Seed=1  SampleTime=0.01
  Random Number5 : RandomNumber  Variance=0.001  Seed=2  SampleTime=0.01
  Random Number6 : RandomNumber  Variance=0.000001  Seed=3  SampleTime=0.01
  IMU : Outport
  wires:
  Random Number2/1 -> ?
  Gain4/1 -> Add3/1
  Cs/1 -> Demux/1
  Add/1 -> Gain4/1
  Demux/1 -> Add/2
  Demux/2 -> Add1/2
  Add1/1 -> Gain1/1
  Random Number1/1 -> ?
  Gain1/1 -> Add4/1
  Mux/1 -> IMU/1
  Demux/3 -> Add2/2
  Add2/1 -> Gain2/1
  Random Number3/1 -> ?
  Add3/1 -> Mux/1
  Random Number4/1 -> Add3/2
  Random Number5/1 -> Add4/2
  Add4/1 -> Mux/2
  Random Number6/1 -> Add5/2
  Gain2/1 -> Add5/1
  Add5/1 -> Mux/3

== system ABS_CHO/Vehicle/Vehicle States (True)/Subsystem2 ==
  note: [rad/s]
  Cs : Inport
  Add2 : Sum
  Gain : Gain  Gain=2*pi/60
  Random Number1 : RandomNumber  Variance=0.00028  SampleTime=0.01
  w_whl : Outport
  wires:
  Cs/1 -> Gain/1
  Add2/1 -> w_whl/1
  Gain/1 -> Add2/2
  Random Number1/1 -> Add2/1

== system ABS_CHO/Vehicle/Vehicle States (True)/Subsystem3 ==
  note: [m/s]
  w : Inport
  Data Store Read : DataStoreRead  DataStoreName=r_e  IndexOptions=Index vector (dialog)  Indices=1  OutputSizes=1
  Product : Product
  v_whl : Outport
  wires:
  w/1 -> Product/2
  Product/1 -> v_whl/1
  Data Store Read/1 -> Product/1

== system ABS_CHO/Vehicle/Vehicle States (True)/Subsystem5 ==
  note: [rad]
  Cs : Inport
  Gain : Gain  Gain=pi/180
  steer : Outport
  wires:
  Cs/1 -> Gain/1
  Gain/1 -> steer/1

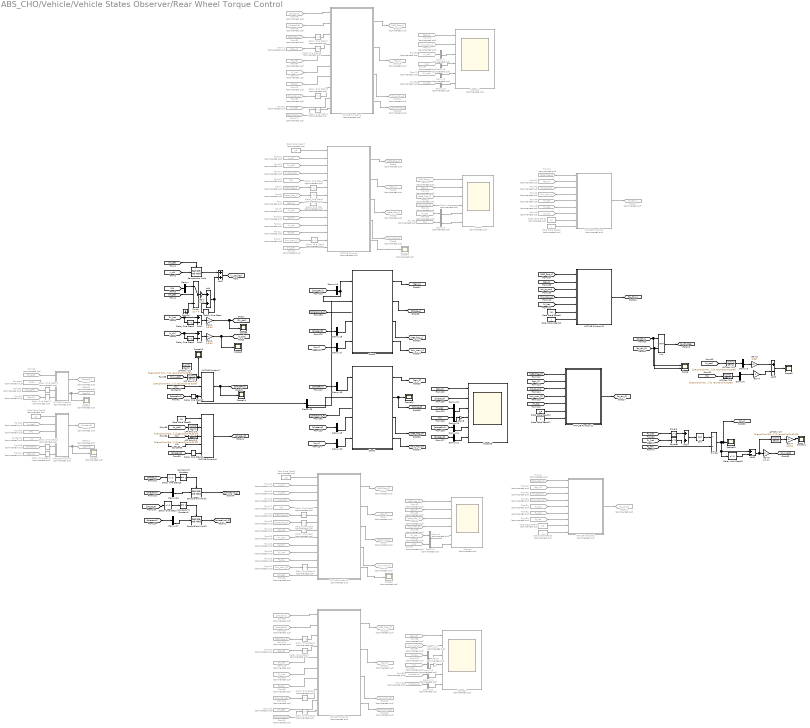
== system ABS_CHO/Vehicle/Vehicle States Observer/Rear Wheel Torque Control ==
  Add : Sum
  Add{1..3,5} (4 alike) : Sum  Inputs=+-
  Add4 : Sum
  Add7 : Sum
  Chart1 : Stateflow chart  TreatAsAtomicUnit=on
      settings: PortSchema="{\"entries\":[{\"content\":{\"sides\":[{\"content\":{\"connectorIds\":[\"In1\",\"In4\",\"In2\",\"In3\"]},\"type\":\"ConnectorPlacement.EquallySpacedRectSide\",\"uuid\":\"db710ea1-fb24-4b0b-941f-cf8c75f21c99\"},{\"content\":{\"connectorIds\":[\"Out1\",\"Out2\",\"Out3\",\"Out4\"],\"side\":\"RIGHT\"},\"type\":\"ConnectorPlacement.EquallySpacedRectSide\",\"uuid\":\"7a28eb5b-b11f-4670-843b-33af1bb3f699\"},{\"content\":{\"side\":\"TOP\"},\"type\":\"ConnectorPlacement.EquallySpacedRectSide\",\"uuid\":\"93d825f3-ffdf-4844-a2ed-a3f99ed38bae\"}]},\"type\":\"ConnectorPlacement.EquallySpacedConnector\",\"uuid\":\"81577ebc-9413-41bd-bf82-8b03e2b63e1f\"}],\"packageUris\":[\"http://schema.mathworks.com/mf0/Connector/R2020b\"],\"version\":\"1.0\"}"
  Chart2 : Stateflow chart  TreatAsAtomicUnit=on
      settings: PortSchema="{\"entries\":[{\"content\":{\"sides\":[{\"content\":{\"connectorIds\":[\"In1\",\"In4\",\"In2\",\"In3\"]},\"type\":\"ConnectorPlacement.EquallySpacedRectSide\",\"uuid\":\"db710ea1-fb24-4b0b-941f-cf8c75f21c99\"},{\"content\":{\"connectorIds\":[\"Out1\",\"Out2\",\"Out3\",\"Out4\"],\"side\":\"RIGHT\"},\"type\":\"ConnectorPlacement.EquallySpacedRectSide\",\"uuid\":\"7a28eb5b-b11f-4670-843b-33af1bb3f699\"},{\"content\":{\"side\":\"TOP\"},\"type\":\"ConnectorPlacement.EquallySpacedRectSide\",\"uuid\":\"93d825f3-ffdf-4844-a2ed-a3f99ed38bae\"}]},\"type\":\"ConnectorPlacement.EquallySpacedConnector\",\"uuid\":\"81577ebc-9413-41bd-bf82-8b03e2b63e1f\"}],\"packageUris\":[\"http://schema.mathworks.com/mf0/Connector/R2020b\"],\"version\":\"1.0\"}"
  Compare To Constant : simulink/Logic and Bit Operations/Compare To Constant  relop===  const=1  OutDataTypeStr=boolean
  Compare To Constant1 : simulink/Logic and Bit Operations/Compare To Constant  relop===  const=1  OutDataTypeStr=boolean
  Constant : Constant  Commented=on  Value=2000
  Constant1 : Constant  Commented=on  Value=10
  Constant2 : Constant  Value=0.1
  Constant3 : Constant  Value=0.5
  Data Store Read{1..2,4,6..7} (5 alike) : DataStoreRead  Commented=on  DataStoreName=r_e  IndexOptions=Index vector (dialog)  Indices=1  OutputSizes=1
  Data Store Read10 : DataStoreRead  DataStoreName=J  IndexOptions=Index vector (dialog)  Indices=1  OutputSizes=1
  Data Store Read11 : DataStoreRead  DataStoreName=J  IndexOptions=Index vector (dialog)  Indices=1  OutputSizes=1
  Data Store Read12 : DataStoreRead  DataStoreName=r_e  IndexOptions=Index vector (dialog)  Indices=1  OutputSizes=1
  Data Store Read3 : DataStoreRead  Commented=on  DataStoreName=J  IndexOptions=Index vector (dialog)  Indices=1  OutputSizes=1
  Data Store Read5 : DataStoreRead  Commented=on  DataStoreName=J  IndexOptions=Index vector (dialog)  Indices=1  OutputSizes=1
  Data Store Read8 : DataStoreRead  DataStoreName=r_e  IndexOptions=Index vector (dialog)  Indices=1  OutputSizes=1
  Data Store Read9 : DataStoreRead  DataStoreName=r_e  IndexOptions=Index vector (dialog)  Indices=1  OutputSizes=1
  Delay One Step : Delay  Commented=on  DelayLength=1  InitialCondition=1  SampleTime=0.01
  Delay One Step{1..3,8..10,16..19,21,23..25} (14 alike) : Delay  Commented=on  DelayLength=1  InitialCondition=0  SampleTime=0.01
  Delay One Step{11..14} (4 alike) : Delay  Commented=on  DelayLength=1  InitialCondition=zeros(4,1)  SampleTime=0.01
  Delay One Step{4..6,15} (4 alike) : Delay  DelayLength=1  SampleTime=0.01
  Delay One Step20 : Delay  DelayLength=1  InitialCondition=zeros(4,1)  SampleTime=0.01
  Delay One Step22 : Delay  DelayLength=1  InitialCondition=zeros(4,1)  SampleTime=0.01
  Delay One Step26 : Delay  DelayLength=1
  Delay One Step27 : Delay  DelayLength=1
  Delay One Step7 : Delay  Commented=on  DelayLength=1  InitialCondition=1  SampleTime=0.01
  Demux : Demux  Outputs=3
  Demux{1..4,7..14} (12 alike) : Demux  Commented=on
  Demux{5,15..27} (14 alike) : Demux
  Demux6 : Demux  Outputs=3
  Divide : Product  Inputs=*/
  From{,18,41,72,76} (5 alike) : From  Commented=on  GotoTag=sgn_L
  From10 : From  Commented=on  GotoTag=sgnFx
  From100 : From  Commented=on  GotoTag=phaseFxd
  From{31,35,50,97,101} (5 alike) : From  Commented=on  GotoTag=mu_max_R
  From{24,36,81,102} (4 alike) : From  Commented=on  GotoTag=brk_stat  TagVisibility=global
  From{9,39,44,51,56,58,83..84,103,118} (10 alike) : From  Commented=on  GotoTag=Fx_hat  TagVisibility=global
  From104 : From  Commented=on  GotoTag=ABS_flag_R
  From{57,59,87,105} (4 alike) : From  Commented=on  GotoTag=slip  TagVisibility=global
  From{66,78,99,106} (4 alike) : From  Commented=on  GotoTag=phasewd
  From{11,25,45,52,74,95} (6 alike) : From  Commented=on  GotoTag=Fy_hat  TagVisibility=global
  From117 : From  Commented=on  GotoTag=zerophase_L
  From{12,26,46,53,75,98} (6 alike) : From  Commented=on  GotoTag=Fz_hat  TagVisibility=global
  From13 : From  Commented=on  GotoTag=IMU  TagVisibility=global
  From14 : From  Commented=on  GotoTag=v_car_hat
  From{15,29,65,90} (4 alike) : From  Commented=on  GotoTag=w_dot
  From16 : From  Commented=on  GotoTag=w_whl  TagVisibility=global
  From{17,21,43,77,80} (5 alike) : From  Commented=on  GotoTag=mu_max_L
  From19 : From  Commented=on  GotoTag=ABS_flag_L
  From20 : From  Commented=on  GotoTag=case_flag_L
  From{22,32,48,94,96} (5 alike) : From  Commented=on  GotoTag=sgn_R
  From23 : From  Commented=on  GotoTag=sgnFx
  From27 : From  Commented=on  GotoTag=IMU  TagVisibility=global
  From28 : From  Commented=on  GotoTag=v_car_hat
  From30 : From  Commented=on  GotoTag=w_whl  TagVisibility=global
  From33 : From  Commented=on  GotoTag=ABS_flag_R
  From34 : From  Commented=on  GotoTag=case_flag_R
  From37 : From  Commented=on  GotoTag=ABS_flag_R
  From38 : From  Commented=on  GotoTag=case_flag_R
  From40 : From  Commented=on  GotoTag=case_flag_L
  From42 : From  Commented=on  GotoTag=brk_tq_cmd  TagVisibility=global
  From47 : From  Commented=on  GotoTag=case_flag_R
  From49 : From  Commented=on  GotoTag=brk_tq_cmd  TagVisibility=global
  From62 : From  Commented=on  GotoTag=Fx_dot
  From63 : From  Commented=on  GotoTag=IMU  TagVisibility=global
  From64 : From  Commented=on  GotoTag=sgnFx
  From67 : From  Commented=on  GotoTag=sgnwd
  From68 : From  Commented=on  GotoTag=phaseFx
  From7 : From  Commented=on  GotoTag=ABS_flag_L
  From73 : From  Commented=on  GotoTag=Fx_dot
  From79 : From  Commented=on  GotoTag=phaseFxd
  From8 : From  Commented=on  GotoTag=case_flag_L
  From82 : From  Commented=on  GotoTag=ABS_flag_L
  From92 : From  Commented=on  GotoTag=zerophase_R
  From93 : From  Commented=on  GotoTag=phaseFxd
  Gain : Gain  Gain=0.01
  Gain{1..2,6..7} (4 alike) : Gain  Gain=1/0.01
  Gain3 : Gain  Gain=0.347
  Gain4 : Gain
  Gain5 : Gain  Commented=on  Gain=-1
  Gain8 : Gain  Gain=-1
  Goto10 : Goto  Commented=on  GotoTag=mu_max_R
  Goto11 : Goto  Commented=on  GotoTag=tq_ctrl_L
  Goto12 : Goto  Commented=on  GotoTag=tq_ctrl_R
  Goto14 : Goto  Commented=on  GotoTag=phaseFx
  Goto15 : Goto  Commented=on  GotoTag=sgnFx
  Goto16 : Goto  Commented=on  GotoTag=phasewd
  Goto17 : Goto  Commented=on  GotoTag=sgnwd
  Goto18 : Goto  Commented=on  GotoTag=sgn_L
  Goto19 : Goto  Commented=on  GotoTag=ABS_flag_L
  Goto20 : Goto  Commented=on  GotoTag=sgn_R
  Goto21 : Goto  Commented=on  GotoTag=mu_max_L
  Goto23 : Goto  Commented=on  GotoTag=ABS_flag_R
  Goto25 : Goto  Commented=on  GotoTag=mu_max_R
  Goto28 : Goto  Commented=on  GotoTag=zerophase_L
  Goto29 : Goto  Commented=on  GotoTag=zerophase_R
  Goto3 : Goto  Commented=on  GotoTag=sgn_L
  Goto4 : Goto  Commented=on  GotoTag=ABS_flag_L
  Goto5 : Goto  Commented=on  GotoTag=case_flag_L
  Goto6 : Goto  Commented=on  GotoTag=mu_max_L
  Goto7 : Goto  Commented=on  GotoTag=sgn_R
  Goto8 : Goto  Commented=on  GotoTag=ABS_flag_R
  Goto9 : Goto  Commented=on  GotoTag=case_flag_R
  Ground : Ground
  LPF 5Hz (1){1..7} (7 alike) : DiscreteFilter  Numerator=[1-exp(-2*pi*0.01*5)]  Denominator=[1 -exp(-2*pi*0.01*5)]  SampleTime=0.01
  MATLAB Function : MATLAB Function  Commented=on  TreatAsAtomicUnit=on
  MATLAB Function1 : MATLAB Function  Commented=on  TreatAsAtomicUnit=on
  MATLAB Function10 : MATLAB Function  TreatAsAtomicUnit=on
  MATLAB Function11 : MATLAB Function  TreatAsAtomicUnit=on
  MATLAB Function2 : MATLAB Function  Commented=on  TreatAsAtomicUnit=on
  MATLAB Function3 : MATLAB Function  Commented=on  TreatAsAtomicUnit=on
  MATLAB Function4 : MATLAB Function  Commented=on  TreatAsAtomicUnit=on
  MATLAB Function5 : MATLAB Function  Commented=on  TreatAsAtomicUnit=on
  MATLAB Function6 : MATLAB Function  Commented=on  TreatAsAtomicUnit=on
  MATLAB Function7 : MATLAB Function  TreatAsAtomicUnit=on
  MATLAB Function8 : MATLAB Function  TreatAsAtomicUnit=on
  MATLAB Function9 : MATLAB Function  Commented=on  TreatAsAtomicUnit=on
  Min : MinMax  Inputs=2
  Sample and Hold : dspsigops/Sample and Hold  trig=Rising edge  initCond=0  latchinput=off
  Sample and Hold1 : dspsigops/Sample and Hold  trig=Rising edge  initCond=0  latchinput=off
  Sample and Hold2 : dspsigops/Sample and Hold  trig=Rising edge  initCond=0  latchinput=off
  Scope : Scope  NumInputPorts=2
  Scope{1,3,12..13} (4 alike) : Scope  Commented=on  NumInputPorts=6
  Scope{5..6,8,10,14..16} (7 alike) : Scope
  Scope11 : Scope  NumInputPorts=2
  Scope18 : Scope  NumInputPorts=6
  Scope{2,4,7,9} (4 alike) : Scope  Commented=on
  Sqrt : Sqrt
  Square : Math  Operator=square
  Square1 : Math  Operator=square
  Switch : Switch  Criteria=u2 > Threshold  SaturateOnIntegerOverflow=off  InputSameDT=off
  tag scope: tq_ctrl_Rear=global
  wires:
  [brk_stat] -> Sample and Hold/Trigger
  [v_whl] -> Sample and Hold/1
  Sample and Hold/1 -> Add7/1
  [IMU] -> Demux/1
  Demux/1 -> Switch/1
  [brk_stat] -> Switch/2
  Ground/1 -> Switch/3
  Switch/1 -> Gain/1
  Add/1 -> Add7/2, Delay One Step4/1
  Add7/1 -> [v_car_hat]
  Add1/1 -> Gain1/1
  MATLAB Function/4(mu_max) -> Goto6/1
  MATLAB Function/2(sgn) -> Goto3/1
  MATLAB Function/3(case_flag) -> Goto5/1
  MATLAB Function/1(ABS_flag) -> Goto4/1
  From/1 -> Delay One Step/1
  Delay One Step/1 -> MATLAB Function/8(sgn_)
  From7/1 -> Delay One Step1/1
  Delay One Step1/1 -> MATLAB Function/6("ABS_flag ")
  From8/1 -> Delay One Step2/1
  Delay One Step2/1 -> MATLAB Function/7("case_flag ")
  From10/1 -> MATLAB Function/10(Fxdot)
  From11/1 -> MATLAB Function/11(Fy)
  From12/1 -> MATLAB Function/12(Fz)
  From14/1 -> MATLAB Function/4(V_hat)
  From15/1 -> MATLAB Function/3(wdot)
  From16/1 -> MATLAB Function/2(w)
  Data Store Read7/1 -> MATLAB Function/1(r_e)
  From17/1 -> Delay One Step3/1
  Delay One Step3/1 -> MATLAB Function/13("mu_max ")
  From18/1 -> Scope1/2  "sgn"
  From20/1 -> Scope1/3  "case"
  From21/1 -> Scope1/4  "mu"
  From19/1 -> Scope1/1  "ABS"
  From24/1 -> MATLAB Function/14(brk_stat)
  [Fx_hat] -> Delay One Step5/1, Add1/1
  From9/1 -> MATLAB Function/9(Fx)
  Delay One Step4/1 -> Add/2
  Gain/1 -> Add/1
  Delay One Step5/1 -> Add1/2
  Delay One Step6/1 -> Add2/2
  [w_whl] -> Delay One Step6/1, Add2/1
  Add2/1 -> Gain2/1
  Delay One Step9/1 -> MATLAB Function1/7("case_flag ")
  From22/1 -> Delay One Step7/1
  From31/1 -> Delay One Step10/1
  MATLAB Function1/3(case_flag) -> Goto9/1
  Delay One Step7/1 -> MATLAB Function1/8(sgn_)
  MATLAB Function1/4(mu_max) -> Goto10/1
  From39/1 -> MATLAB Function1/9(Fx)
  From28/1 -> MATLAB Function1/4(V_hat)
  MATLAB Function1/2(sgn) -> Goto7/1
  From38/1 -> Delay One Step9/1
  From26/1 -> MATLAB Function1/12(Fz)
  From25/1 -> MATLAB Function1/11(Fy)
  From23/1 -> MATLAB Function1/10(Fxdot)
  From34/1 -> Scope3/3  "case"
  From33/1 -> Scope3/1  "ABS"
  From37/1 -> Delay One Step8/1
  MATLAB Function1/1(ABS_flag) -> Goto8/1
  Data Store Read1/1 -> MATLAB Function1/1(r_e)
  From35/1 -> Scope3/4  "mu"
  From29/1 -> MATLAB Function1/3(wdot)
  From30/1 -> MATLAB Function1/2(w)
  From32/1 -> Scope3/2  "sgn"
  Delay One Step10/1 -> MATLAB Function1/13("mu_max ")
  From36/1 -> MATLAB Function1/14(brk_stat)
  Delay One Step8/1 -> MATLAB Function1/6("ABS_flag ")
  Data Store Read2/1 -> MATLAB Function2/8(r_e)
  Data Store Read3/1 -> MATLAB Function2/9(J)
  From40/1 -> MATLAB Function2/1(case_flag)  "case"
  From41/1 -> MATLAB Function2/2(sgn)  "sgn"
  From42/1 -> MATLAB Function2/3(tq_cmd)
  From43/1 -> MATLAB Function2/4(mu_max)  "mu"
  From44/1 -> MATLAB Function2/5(Fx)
  From45/1 -> MATLAB Function2/6(Fy)
  From46/1 -> MATLAB Function2/7(Fz)
  MATLAB Function2/1(tq_out) -> Goto11/1
  From50/1 -> MATLAB Function3/4(mu_max)  "mu"
  From52/1 -> MATLAB Function3/6(Fy)
  From53/1 -> MATLAB Function3/7(Fz)
  From47/1 -> MATLAB Function3/1(case_flag)  "case"
  Data Store Read5/1 -> MATLAB Function3/9(J)
  From48/1 -> MATLAB Function3/2(sgn)  "sgn"
  From51/1 -> MATLAB Function3/5(Fx)
  From49/1 -> MATLAB Function3/3(tq_cmd)
  Data Store Read4/1 -> MATLAB Function3/8(r_e)
  MATLAB Function3/1(tq_out) -> Goto12/1
  [tq_ctrl_R] -> Scope/2, Min/2  "R"
  [tq_ctrl_L] -> Scope/1, Min/1  "L"
  Min/1 -> [tq_ctrl_Rear]
  MATLAB Function1/5(a) -> Scope2/1
  MATLAB Function/5(a) -> Scope4/1
  Gain2/1 -> Scope8/1, [w_dot]
  From13/1 -> MATLAB Function/5(IMU)
  From27/1 -> MATLAB Function1/5(IMU)
  From56/1 -> Demux1/1
  Demux1/4 -> Scope3/5  "Fx"
  From57/1 -> Demux2/1
  Demux2/4 -> Scope3/6  "slip"
  From59/1 -> Demux4/1
  Demux4/3 -> Scope1/6  "slip"
  Demux3/3 -> Scope1/5  "Fx"
  From58/1 -> Demux3/1
  Demux5/3 -> Gain3/1
  Gain3/1 -> Add3/1
  Demux6/1 -> Gain4/1
  Gain4/1 -> Add3/2
  Add3/1 -> Scope5/1
  Gain1/1 -> [Fx_dot], Scope6/1
  Constant/1 -> MATLAB Function4/2(thrs)
  MATLAB Function4/1(phase) -> Goto14/1
  From68/1 -> Delay One Step11/1
  Delay One Step11/1 -> MATLAB Function4/3("phase ")
  MATLAB Function4/2(sgn) -> Scope7/1, Goto15/1
  Delay One Step12/1 -> MATLAB Function4/4("sgn ")
  From64/1 -> Delay One Step12/1
  From62/1 -> MATLAB Function4/1(u)
  MATLAB Function5/1(phase) -> Goto16/1
  Delay One Step14/1 -> MATLAB Function5/6("sgn ")
  MATLAB Function5/2(sgn) -> Scope9/1, Goto17/1
  Constant1/1 -> MATLAB Function5/4(thrs)
  Delay One Step13/1 -> MATLAB Function5/5("phase ")
  From67/1 -> Delay One Step14/1
  From66/1 -> Delay One Step13/1
  From65/1 -> MATLAB Function5/2(u)
  Data Store Read6/1 -> MATLAB Function5/1(r_e)
  From63/1 -> MATLAB Function5/3(IMU)
  [Fx_hat] -> Square/1
  [Fy_hat] -> Square1/1
  Square/1 -> Add4/1
  Square1/1 -> ?
  Add4/1 -> Sqrt/1
  Sqrt/1 -> Divide/1
  [Fz_hat] -> Divide/2
  Divide/1 -> Delay One Step15/1, Add5/1, [mux], Scope10/1
  Delay One Step15/1 -> Add5/2
  From75/1 -> MATLAB Function6/7(Fz)
  From81/1 -> MATLAB Function6/9(brk_stat)
  MATLAB Function6/1(ABS_flag) -> Goto19/1
  From72/1 -> Delay One Step16/1
  From74/1 -> MATLAB Function6/6(Fy)
  From84/1 -> MATLAB Function6/5(Fx)
  From78/1 -> MATLAB Function6/1(phasewd)
  From82/1 -> Delay One Step17/1
  From80/1 -> Delay One Step19/1
  MATLAB Function6/3(mu_max) -> Goto21/1
  Delay One Step19/1 -> MATLAB Function6/8("mu_max ")
  Delay One Step17/1 -> MATLAB Function6/3("ABS_flag ")
  Delay One Step16/1 -> MATLAB Function6/4(sgn_)
  MATLAB Function6/2(sgn) -> Goto18/1
  [phaseFxd] -> Delay One Step20/1
  Delay One Step22/1 -> MATLAB Function8/5("phase ")
  Constant3/1 -> MATLAB Function8/4(thrs)
  [phasewd] -> Delay One Step22/1
  Delay One Step20/1 -> Demux25/1, MATLAB Function7/3("phase ")
  Data Store Read9/1 -> MATLAB Function8/1(r_e)
  Constant2/1 -> MATLAB Function7/2(thrs)
  From79/1 -> MATLAB Function6/2(phaseFxd)
  From76/1 -> Scope12/1  "sgn"
  From77/1 -> Scope12/2  "mu"
  From83/1 -> Demux7/1
  From87/1 -> Demux8/1
  Demux7/3 -> Scope12/3  "Fx"
  Demux8/3 -> Scope12/4  "slip"
  From73/1 -> Demux9/1
  Demux9/3 -> Scope12/5  "Fxd"
  From90/1 -> Demux10/1
  Demux10/3 -> Scope12/6  "wd"
  From105/1 -> Demux13/1
  Demux11/4 -> Scope13/6  "wd"
  From103/1 -> Demux12/1
  From97/1 -> Scope13/2  "mu"
  Demux14/4 -> Scope13/5  "Fxd"
  From93/1 -> Demux14/1
  Demux12/4 -> Scope13/3  "Fx"
  Demux13/4 -> Gain5/1  "slip"
  From96/1 -> Scope13/1  "sgn"
  From106/1 -> Demux11/1
  [sgn_L] -> MATLAB Function10/2(sgn)  "sgn"
  Data Store Read8/1 -> MATLAB Function10/6(r_e)
  MATLAB Function10/1(tq_out) -> [tq_ctrl_L]
  [ABS_flag_L] -> MATLAB Function10/1(ABS_flag)  "ABS"
  [mu_max_L] -> MATLAB Function10/4(mu_max)  "mu"
  [Fx_hat] -> MATLAB Function10/5(Fx)
  [brk_tq_cmd] -> MATLAB Function10/3(tq_cmd)
  Data Store Read10/1 -> MATLAB Function10/7(J)
  [Fx_hat] -> MATLAB Function11/5(Fx)
  [mu_max_R] -> MATLAB Function11/4(mu_max)  "mu"
  [brk_tq_cmd] -> MATLAB Function11/3(tq_cmd)
  [ABS_flag_R] -> MATLAB Function11/1(ABS_flag)  "ABS"
  MATLAB Function11/1(tq_out) -> [tq_ctrl_R]
  Data Store Read11/1 -> MATLAB Function11/7(J)
  Data Store Read12/1 -> MATLAB Function11/6(r_e)
  [sgn_R] -> MATLAB Function11/2(sgn)  "sgn"
  MATLAB Function6/4(zerophase) -> Goto28/1
  Delay One Step24/1 -> MATLAB Function6/10("zerophase ")
  From117/1 -> Delay One Step24/1
  Gain5/1 -> Scope13/4  "slip"
  MATLAB Function7/1(phase) -> Scope14/1, [phaseFxd]
  MATLAB Function8/1(phase) -> [phasewd]
  [w_dot] -> LPF 5Hz (1)4/1
  [IMU] -> LPF 5Hz (1)5/1
  Add5/1 -> LPF 5Hz (1)7/1, Gain6/1
  Gain6/1 -> [mux_dot]
  LPF 5Hz (1)7/1 -> Gain7/1
  Gain7/1 -> Scope11/1
  From104/1 -> Delay One Step21/1
  From95/1 -> MATLAB Function9/6(Fy)
  From99/1 -> MATLAB Function9/1(phasewd)
  Delay One Step25/1 -> MATLAB Function9/10("zerophase ")
  MATLAB Function9/4(zerophase) -> Goto29/1
  From92/1 -> Delay One Step25/1
  Delay One Step21/1 -> MATLAB Function9/3("ABS_flag ")
  From98/1 -> MATLAB Function9/7(Fz)
  From102/1 -> MATLAB Function9/9(brk_stat)
  From100/1 -> MATLAB Function9/2(phaseFxd)
  MATLAB Function9/2(sgn) -> Goto20/1
  From101/1 -> Delay One Step23/1
  Delay One Step18/1 -> MATLAB Function9/4(sgn_)
  From94/1 -> Delay One Step18/1
  MATLAB Function9/1(ABS_flag) -> Goto23/1
  MATLAB Function9/3(mu_max) -> Goto25/1
  Delay One Step23/1 -> MATLAB Function9/8("mu_max ")
  From118/1 -> MATLAB Function9/5(Fx)
  LPF 5Hz (1)4/1 -> Demux5/1
  LPF 5Hz (1)5/1 -> Demux6/1
  [phaseFxd] -> Demux15/1
  [phasewd] -> Demux16/1
  Chart2/1(sgn) -> [sgn_L]
  Demux15/3 -> Chart2/1(Fxd)
  Demux16/3 -> Chart2/2(wd)
  Chart2/2(phase) -> [phase_L]
  Chart2/3(ABS_flag) -> [ABS_flag_L]
  [mux] -> Demux17/1
  Demux17/3 -> Chart2/3(mu)
  Chart2/4(mu_max) -> [mu_max_L]
  Demux20/4 -> Chart1/3(mu)
  Demux19/4 -> Chart1/2(wd)
  [mux] -> Demux20/1
  Chart1/3(ABS_flag) -> [ABS_flag_R]
  [phaseFxd] -> Demux18/1
  Chart1/2(phase) -> Scope16/1, [phase_R]
  [phasewd] -> Demux19/1
  Demux18/4 -> Chart1/1(Fxd)
  Chart1/4(mu_max) -> [mu_max_R]
  Chart1/1(sgn) -> [sgn_R]
  Gain8/1 -> Scope18/4  "slip"
  [slip] -> Demux23/1
  Demux21/4 -> Scope18/6  "wd"
  Demux23/4 -> Gain8/1  "slip"
  Demux22/4 -> Scope18/3  "Fx"
  [phasewd] -> Demux21/1
  [phaseFxd] -> Demux24/1
  [phase_R] -> Scope18/2  "phase"
  Demux24/4 -> Scope18/5  "Fxd"
  [Fx_hat] -> Demux22/1
  [sgn_R] -> Scope18/1  "sgn"
  Demux25/4 -> Chart1/4(Fxd_)
  Demux25/3 -> Chart2/4(Fxd_)
  [w_dot] -> LPF 5Hz (1)3/1
  [IMU] -> LPF 5Hz (1)6/1
  [mux_dot] -> LPF 5Hz (1)1/1
  [phase_L] -> Delay One Step26/1
  Compare To Constant/1 -> Sample and Hold1/Trigger
  [phasewd] -> Demux26/1
  Sample and Hold1/1 -> [phase1wd_L]
  Demux26/3 -> Sample and Hold1/1
  Demux27/4 -> Sample and Hold2/1
  Compare To Constant1/1 -> Sample and Hold2/Trigger
  [phasewd] -> Demux27/1
  [phase_R] -> Delay One Step27/1
  Sample and Hold2/1 -> [phase1wd_R]
  [phase1wd_L] -> ?
  [phase1wd_R] -> ?
  Delay One Step26/1 -> Compare To Constant/1
  Delay One Step27/1 -> Compare To Constant1/1
  LPF 5Hz (1)1/1 -> Scope15/1, MATLAB Function7/1(u)
  LPF 5Hz (1)3/1 -> MATLAB Function8/2(u)
  LPF 5Hz (1)6/1 -> MATLAB Function8/3(IMU)
